simulink model "Furuta_Control_mbed"  (R2017a)
settings: Solver=FixedStepDiscrete  StartTime=0.0  StopTime=3  FixedStep=Ts  RelTol=1e-3
PreLoadFcn:
  | %myBusDef
StartFcn:
  | % Full path to the block
  | %blk = 'Furuta_Control/Bus Creator';
  | 
  | % Attach the event listener
  | %h = add_exec_event_listener(blk, ...
  | %         'PostOutputs', @displayBusdata);
values from neighbouring files (symbols this model uses):
  K = Pxy*pinv(Pyy)    [UKF_RECURSIVE.m]    (also in example2.m = P12inv(P2); exemple_statler.m = Pxy/Pyy; exemple_statler2.m = Pxy/Pyy; ukf_teste.m = Pxy/Pyy)
settings Model: Creator=Marcelo  LastModifiedBy=felip
settings SolverCC: ZeroCrossControl=DisableAll
settings OptimizationCC: DefaultParameterBehavior=Inlined  UseDivisionForNetSlopeComputation=on  UseFloatMulNetSlope=on  InlineInvariantSignals=on  PassReuseOutputArgsAs=Individual arguments  ZeroExternalMemoryAtStartup=off  ZeroInternalMemoryAtStartup=off  NoFixptDivByZeroProtection=on  EfficientFloat2IntCast=on  LifeSpan=1
settings DebuggingCC: ParameterOverflowMsg=warning  ParameterTunabilityLossMsg=error  BusObjectLabelMismatch=error
settings HardwareCC: ProdBitPerPointer=32  ProdBitPerSizeT=32  ProdBitPerPtrDiffT=32  ProdLargestAtomicInteger=Long  ProdLargestAtomicFloat=Double  ProdWordSize=32  ProdHWDeviceType=ARM Compatible->ARM Cortex
settings ModelReferenceCC: ModelReferenceMinAlgLoopOccurrences=on
settings SFSimCC: MATLABDynamicMemAlloc=off
settings RTWCC: SystemTargetFile=ert.tlc  TemplateMakefile=ert_default_tmf  Description=Embedded Coder  GenerateReport=on  IncludeHyperlinkInReport=on  LaunchReport=on  GenerateTraceInfo=on  GenerateTraceReport=on  GenerateTraceReportSl=on  GenerateTraceReportSf=on  GenerateTraceReportEml=on  GenerateCodeMetricsReport=on
settings CodeAppCC: ForceParamTrailComments=on  IgnoreCustomStorageClasses=off  OperatorAnnotations=on  SimulinkDataObjDesc=on  SFDataObjDesc=on  MATLABFcnDesc=on  CustomSymbolStrGlobalVar=rt$N$M  CustomSymbolStrType=$N$M  CustomSymbolStrFcn=$N$M$F  CustomSymbolStrMacro=$N$M  InsertBlockDesc=on  MATLABSourceComments=on
settings ERTTargetCC: TargetLangStandard=C99 (ISO)  GenerateSampleERTMain=on  IncludeMdlTerminateFcn=off  CombineSignalStateStructs=on  SuppressErrorStatus=on  SupportAbsoluteTime=off  SupportComplex=off  InlinedParameterPlacement=NonHierarchical  ERTCustomFileTemplate=example_file_process.tlc  ERTFilePackagingFormat=CompactWithDataFile
settings ConfigComp: PLC_TargetIDE=codesys23  PLC_GenerateReport=off

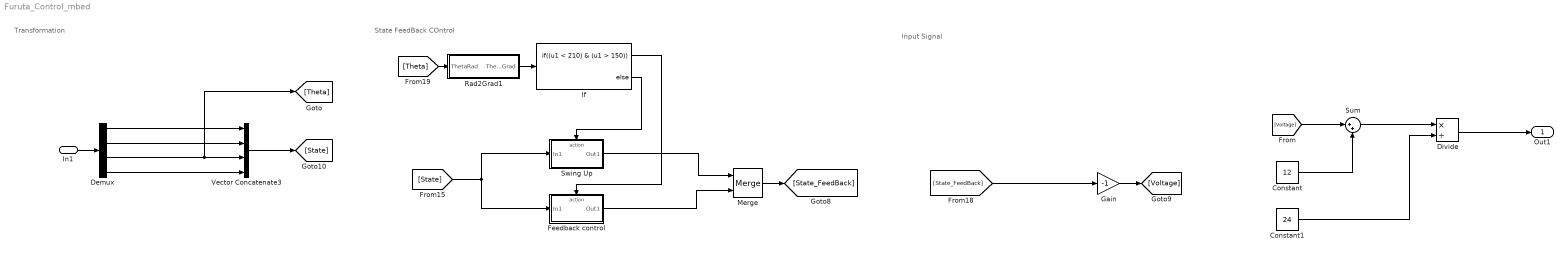
== system Furuta_Control_mbed ==
  note: Transformation
  note: State FeedBack COntrol
  note: Input Signal
  In1 : Inport
  Constant : Constant  Value=12
  Constant1 : Constant  Value=24
  Demux : Demux
  Divide : Product  Inputs=*/
  Feedback control : Subsystem  TreatAsAtomicUnit=on
  Gain : Gain  Gain=-1
  If : If  IfExpression=(u1 < 210) & (u1 > 150)
  Merge : Merge
  Rad2Grad1 : Subsystem
  Sum : Sum  Inputs=|++
  Swing Up : Subsystem  TreatAsAtomicUnit=on
  Vector Concatenate3 : Concatenate  NumInputs=4
  Out1 : Outport
  wires:
  [State_FeedBack] -> Gain/1
  Vector Concatenate3/1 -> [State]
  If/2 -> Swing Up/Action
  [State] -> Feedback control/1(In1), Swing Up/1(In1)
  Swing Up/1(Out1) -> Merge/1
  Merge/1 -> [State_FeedBack]
  If/1 -> Feedback control/Action
  Rad2Grad1/1(ThetaGrad) -> If/1
  [Theta] -> Rad2Grad1/1(ThetaRad)
  Feedback control/1(Out1) -> Merge/2
  Gain/1 -> [Voltage]
  [Voltage] -> Sum/1
  Constant/1 -> Sum/2
  Sum/1 -> Divide/1
  Constant1/1 -> Divide/2
  Divide/1 -> Out1/1
  Demux/2 -> Vector Concatenate3/2
  Demux/3 -> [Theta], Vector Concatenate3/3
  Demux/4 -> Vector Concatenate3/4
  In1/1 -> Demux/1
  Demux/1 -> Vector Concatenate3/1

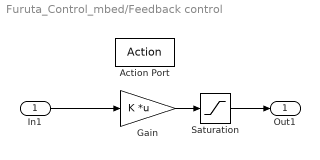
== system Furuta_Control_mbed/Feedback control ==
  In1 : Inport
  Action Port : ActionPort  ActionType=then
  Gain : Gain  Gain=K  Multiplication=Matrix(K*u)  ParamDataTypeStr=double  OutDataTypeStr=double
  Saturation : Saturate  UpperLimit=12  LowerLimit=-12
  Out1 : Outport
  wires:
  In1/1 -> Gain/1
  Gain/1 -> Saturation/1
  Saturation/1 -> Out1/1

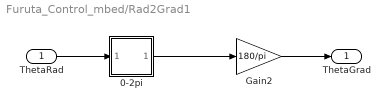
== system Furuta_Control_mbed/Rad2Grad1 ==
  ThetaRad : Inport
  0-2pi : Subsystem
  Gain2 : Gain  Gain=180/pi
  ThetaGrad : Outport
  wires:
  ThetaRad/1 -> 0-2pi/1(In1)
  0-2pi/1(Out1) -> Gain2/1
  Gain2/1 -> ThetaGrad/1

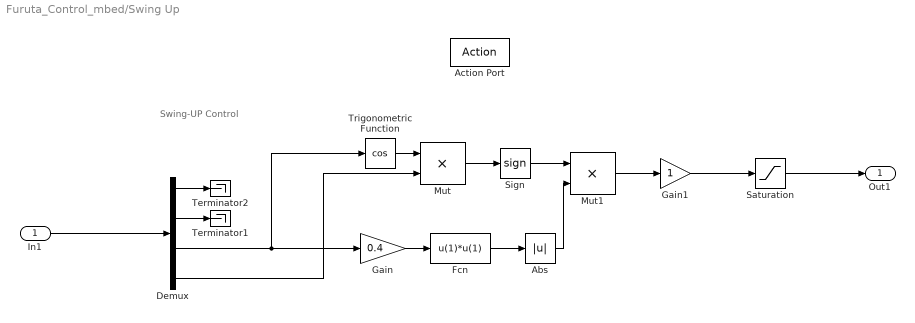
== system Furuta_Control_mbed/Swing Up ==
  note: Swing-UP Control
  In1 : Inport
  Action Port : ActionPort  ActionType=else
  Abs : Abs
  Demux : Demux
  Fcn : Fcn  Expr=u(1)*u(1)
  Gain : Gain  Gain=0.4
  Gain1 : Gain
  Mut : Product  Inputs=**
  Mut1 : Product  Inputs=**
  Saturation : Saturate  UpperLimit=12  LowerLimit=-12
  Sign : Signum
  Terminator1 : Terminator
  Terminator2 : Terminator
  Trigonometric Function : Trigonometry  Operator=cos
  Out1 : Outport  InitialOutput=0
  wires:
  Saturation/1 -> Out1/1
  Demux/2 -> Terminator1/1
  Demux/1 -> Terminator2/1
  Gain1/1 -> Saturation/1
  Mut1/1 -> Gain1/1
  Demux/3 -> Trigonometric Function/1, Gain/1
  Fcn/1 -> Abs/1
  Trigonometric Function/1 -> Mut/1
  Demux/4 -> Mut/2
  Abs/1 -> Mut1/2
  Sign/1 -> Mut1/1
  Mut/1 -> Sign/1
  Gain/1 -> Fcn/1
  In1/1 -> Demux/1

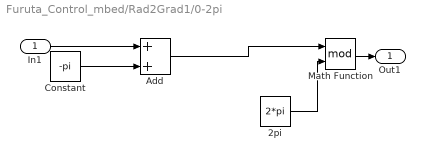
== system Furuta_Control_mbed/Rad2Grad1/0-2pi ==
  In1 : Inport
  2pi : Constant  Value=2*pi
  Add : Sum
  Constant : Constant  Value=-pi
  Math Function : Math  Operator=mod  SaturateOnIntegerOverflow=on
  Out1 : Outport
  wires:
  Math Function/1 -> Out1/1
  2pi/1 -> Math Function/2
  Constant/1 -> Add/2
  In1/1 -> Add/1
  Add/1 -> Math Function/1
